simulink model "CM020A_Bmw5441McuCfg"  (R2013b)
settings: Solver=FixedStepDiscrete  SolverMode=SingleTasking  StartTime=0.0  StopTime=1  FixedStep=0.0005  RelTol=1e-3
PreLoadFcn:
  | CM020A_Bmw5441McuCfg_DataDict
values from neighbouring files (symbols this model uses):
  ADC0CFGANDUSE_ADCD0SGVCEP2_CNT_U08 = DataDict.Constant    [CM020A_Bmw5441McuCfg_DataDict.m]
  ADC0CFGANDUSE_ADCD0SGVCEP3_CNT_U08 = DataDict.Constant    [CM020A_Bmw5441McuCfg_DataDict.m]
  ADC0CFGANDUSE_ADCD0SGVCSP2_CNT_U08 = DataDict.Constant    [CM020A_Bmw5441McuCfg_DataDict.m]
  ADC0CFGANDUSE_ADCD0SGVCSP3_CNT_U08 = DataDict.Constant    [CM020A_Bmw5441McuCfg_DataDict.m]
  ADC0CFGANDUSE_ADCD0VCR00_CNT_U32 = DataDict.Constant    [CM020A_Bmw5441McuCfg_DataDict.m]
  ADC0CFGANDUSE_ADCD0VCR01_CNT_U32 = DataDict.Constant    [CM020A_Bmw5441McuCfg_DataDict.m]
  ADC0CFGANDUSE_ADCD0VCR02_CNT_U32 = DataDict.Constant    [CM020A_Bmw5441McuCfg_DataDict.m]
  ADC0CFGANDUSE_ADCD0VCR03_CNT_U32 = DataDict.Constant    [CM020A_Bmw5441McuCfg_DataDict.m]
  ADC0CFGANDUSE_ADCD0VCR04_CNT_U32 = DataDict.Constant    [CM020A_Bmw5441McuCfg_DataDict.m]
  ADC0CFGANDUSE_ADCD0VCR05_CNT_U32 = DataDict.Constant    [CM020A_Bmw5441McuCfg_DataDict.m]
  ADC0CFGANDUSE_ADCD0VCR06_CNT_U32 = DataDict.Constant    [CM020A_Bmw5441McuCfg_DataDict.m]
  ADC0CFGANDUSE_ADCD0VCR07_CNT_U32 = DataDict.Constant    [CM020A_Bmw5441McuCfg_DataDict.m]
  ADC0CFGANDUSE_ADCD0VCR08_CNT_U32 = DataDict.Constant    [CM020A_Bmw5441McuCfg_DataDict.m]
  ADC0CFGANDUSE_ADCD0VCR09_CNT_U32 = DataDict.Constant    [CM020A_Bmw5441McuCfg_DataDict.m]
  ADC0CFGANDUSE_ADCD0VCR10_CNT_U32 = DataDict.Constant    [CM020A_Bmw5441McuCfg_DataDict.m]
  ADC0CFGANDUSE_ADCD0VCR11_CNT_U32 = DataDict.Constant    [CM020A_Bmw5441McuCfg_DataDict.m]
  ADC0CFGANDUSE_ADCD0VCR12_CNT_U32 = DataDict.Constant    [CM020A_Bmw5441McuCfg_DataDict.m]
  ADC0CFGANDUSE_ADCD0VCR13_CNT_U32 = DataDict.Constant    [CM020A_Bmw5441McuCfg_DataDict.m]
  ADC0CFGANDUSE_ADCD0VCR14_CNT_U32 = DataDict.Constant    [CM020A_Bmw5441McuCfg_DataDict.m]
  ADC0CFGANDUSE_ADCD0VCR15_CNT_U32 = DataDict.Constant    [CM020A_Bmw5441McuCfg_DataDict.m]
  ADC0CFGANDUSE_ADCD0VCR16_CNT_U32 = DataDict.Constant    [CM020A_Bmw5441McuCfg_DataDict.m]
  ADC0CFGANDUSE_ADCD0VCR17_CNT_U32 = DataDict.Constant    [CM020A_Bmw5441McuCfg_DataDict.m]
  ADC0CFGANDUSE_ADCD0VCR18_CNT_U32 = DataDict.Constant    [CM020A_Bmw5441McuCfg_DataDict.m]
  ADC0CFGANDUSE_ADCD0VCR19_CNT_U32 = DataDict.Constant    [CM020A_Bmw5441McuCfg_DataDict.m]
  ADC0CFGANDUSE_ADCD0VCR20_CNT_U32 = DataDict.Constant    [CM020A_Bmw5441McuCfg_DataDict.m]
  ADC0CFGANDUSE_ADCSCAGFAC_VOLTPERCNT_F32 = DataDict.Constant    [CM020A_Bmw5441McuCfg_DataDict.m]
  ADC1CFGANDUSE_ADCD1SGVCEP2_CNT_U08 = DataDict.Constant    [CM020A_Bmw5441McuCfg_DataDict.m]
  ADC1CFGANDUSE_ADCD1SGVCEP3_CNT_U08 = DataDict.Constant    [CM020A_Bmw5441McuCfg_DataDict.m]
  ADC1CFGANDUSE_ADCD1SGVCSP2_CNT_U08 = DataDict.Constant    [CM020A_Bmw5441McuCfg_DataDict.m]
  ADC1CFGANDUSE_ADCD1SGVCSP3_CNT_U08 = DataDict.Constant    [CM020A_Bmw5441McuCfg_DataDict.m]
  ADC1CFGANDUSE_ADCD1VCR00_CNT_U32 = DataDict.Constant    [CM020A_Bmw5441McuCfg_DataDict.m]
  ADC1CFGANDUSE_ADCD1VCR01_CNT_U32 = DataDict.Constant    [CM020A_Bmw5441McuCfg_DataDict.m]
  ADC1CFGANDUSE_ADCD1VCR02_CNT_U32 = DataDict.Constant    [CM020A_Bmw5441McuCfg_DataDict.m]
  ADC1CFGANDUSE_ADCD1VCR03_CNT_U32 = DataDict.Constant    [CM020A_Bmw5441McuCfg_DataDict.m]
  ADC1CFGANDUSE_ADCD1VCR04_CNT_U32 = DataDict.Constant    [CM020A_Bmw5441McuCfg_DataDict.m]
  ADC1CFGANDUSE_ADCD1VCR05_CNT_U32 = DataDict.Constant    [CM020A_Bmw5441McuCfg_DataDict.m]
  ADC1CFGANDUSE_ADCD1VCR06_CNT_U32 = DataDict.Constant    [CM020A_Bmw5441McuCfg_DataDict.m]
  ADC1CFGANDUSE_ADCD1VCR07_CNT_U32 = DataDict.Constant    [CM020A_Bmw5441McuCfg_DataDict.m]
  ADC1CFGANDUSE_ADCD1VCR08_CNT_U32 = DataDict.Constant    [CM020A_Bmw5441McuCfg_DataDict.m]
  ADC1CFGANDUSE_ADCD1VCR09_CNT_U32 = DataDict.Constant    [CM020A_Bmw5441McuCfg_DataDict.m]
  ADC1CFGANDUSE_ADCD1VCR10_CNT_U32 = DataDict.Constant    [CM020A_Bmw5441McuCfg_DataDict.m]
  ADC1CFGANDUSE_ADCD1VCR11_CNT_U32 = DataDict.Constant    [CM020A_Bmw5441McuCfg_DataDict.m]
  ADC1CFGANDUSE_ADCD1VCR12_CNT_U32 = DataDict.Constant    [CM020A_Bmw5441McuCfg_DataDict.m]
  ADC1CFGANDUSE_ADCD1VCR13_CNT_U32 = DataDict.Constant    [CM020A_Bmw5441McuCfg_DataDict.m]
  ADC1CFGANDUSE_ADCD1VCR14_CNT_U32 = DataDict.Constant    [CM020A_Bmw5441McuCfg_DataDict.m]
  ADC1CFGANDUSE_ADCD1VCR15_CNT_U32 = DataDict.Constant    [CM020A_Bmw5441McuCfg_DataDict.m]
  ADC1CFGANDUSE_ADCD1VCR16_CNT_U32 = DataDict.Constant    [CM020A_Bmw5441McuCfg_DataDict.m]
  ADC1CFGANDUSE_ADCD1VCR17_CNT_U32 = DataDict.Constant    [CM020A_Bmw5441McuCfg_DataDict.m]
  ADC1CFGANDUSE_ADCD1VCR18_CNT_U32 = DataDict.Constant    [CM020A_Bmw5441McuCfg_DataDict.m]
  ADC1CFGANDUSE_ADCD1VCR19_CNT_U32 = DataDict.Constant    [CM020A_Bmw5441McuCfg_DataDict.m]
  ADC1CFGANDUSE_ADCD1VCR20_CNT_U32 = DataDict.Constant    [CM020A_Bmw5441McuCfg_DataDict.m]
  ADCDIAGC_DYNDIAGFAILSTEP_CNT_U16 = DataDict.Constant    [CM020A_Bmw5441McuCfg_DataDict.m]
  ADCDIAGC_DYNDIAGPASSSTEP_CNT_U16 = DataDict.Constant    [CM020A_Bmw5441McuCfg_DataDict.m]
  BATTRTNCURR_CURRESTIMDIFTHD_AMPR_F32 = DataDict.Constant    [CM020A_Bmw5441McuCfg_DataDict.m]
  BATTRTNCURR_FAILSTEP_CNT_U16 = DataDict.Constant    [CM020A_Bmw5441McuCfg_DataDict.m]
  BATTRTNCURR_FASTLOOPPROC_CNT_LOGL = DataDict.Constant    [CM020A_Bmw5441McuCfg_DataDict.m]
  BATTRTNCURR_FILCUTFREQ_HZ_F32 = DataDict.Constant    [CM020A_Bmw5441McuCfg_DataDict.m]
  BATTRTNCURR_GAIN_AMPRPERVOLT_F32 = DataDict.Constant    [CM020A_Bmw5441McuCfg_DataDict.m]
  BATTRTNCURR_LOWRTHD_AMPR_F32 = DataDict.Constant    [CM020A_Bmw5441McuCfg_DataDict.m]
  BATTRTNCURR_OFFSET_VOLT_F32 = DataDict.Constant    [CM020A_Bmw5441McuCfg_DataDict.m]
  BATTRTNCURR_OUTPMAX_AMPR_F32 = DataDict.Constant    [CM020A_Bmw5441McuCfg_DataDict.m]
  BATTRTNCURR_OUTPMIN_AMPR_F32 = DataDict.Constant    [CM020A_Bmw5441McuCfg_DataDict.m]
  BATTRTNCURR_PASSSTEP_CNT_U16 = DataDict.Constant    [CM020A_Bmw5441McuCfg_DataDict.m]
  BATTRTNCURR_UPPRTHD_AMPR_F32 = DataDict.Constant    [CM020A_Bmw5441McuCfg_DataDict.m]
  BATTVLTGSCAGFAC_ULS_F32 = DataDict.Constant    [CM020A_Bmw5441McuCfg_DataDict.m]
  BATTVLTGSWD1SCAGFAC_ULS_F32 = DataDict.Constant    [CM020A_Bmw5441McuCfg_DataDict.m]
  ECUTMEAS_DFTT_DEGCGRD_F32 = DataDict.Constant    [CM020A_Bmw5441McuCfg_DataDict.m]
  ECUTMEAS_ECUTX_VOLT_U3P13 = DataDict.Constant    [CM020A_Bmw5441McuCfg_DataDict.m]
  ECUTMEAS_ECUTY_DEGCGRD_S8P7 = DataDict.Constant    [CM020A_Bmw5441McuCfg_DataDict.m]
  ECUTMEAS_FILTAU_HZ_F32 = DataDict.Constant    [CM020A_Bmw5441McuCfg_DataDict.m]
  ECUTMEAS_NTC0X045FAILSTEP_CNT_U16 = DataDict.Constant    [CM020A_Bmw5441McuCfg_DataDict.m]
  ECUTMEAS_NTC0X045PASSSTEP_CNT_U16 = DataDict.Constant    [CM020A_Bmw5441McuCfg_DataDict.m]
  ECUTMEAS_RNGDIAGCMAX_DEGCGRD_F32 = DataDict.Constant    [CM020A_Bmw5441McuCfg_DataDict.m]
  ECUTMEAS_RNGDIAGCMIN_DEGCGRD_F32 = DataDict.Constant    [CM020A_Bmw5441McuCfg_DataDict.m]
  ELECGLBPRM_IVTRCNT_CNT_U08 = DataDict.Constant    [CM020A_Bmw5441McuCfg_DataDict.m]
  ELECGLBPRM_PWMFRQMAX_HZ_U32 = DataDict.Constant    [CM020A_Bmw5441McuCfg_DataDict.m]
  ELECGLBPRM_PWMFRQMIN_HZ_U32 = DataDict.Constant    [CM020A_Bmw5441McuCfg_DataDict.m]
  ELECGLBPRM_PWMPERDMAX_NANOSEC_U32 = DataDict.Constant    [CM020A_Bmw5441McuCfg_DataDict.m]
  ELECGLBPRM_PWMPERDMIN_NANOSEC_U32 = DataDict.Constant    [CM020A_Bmw5441McuCfg_DataDict.m]
  ELECGLBPRM_PWMPERDNOM_MICROSEC_U7P9 = DataDict.Constant    [CM020A_Bmw5441McuCfg_DataDict.m]
  ELECGLBPRM_PWMPERDNOMX2_SEC_F32 = DataDict.Constant    [CM020A_Bmw5441McuCfg_DataDict.m]
  FLTINJENA = DataDict.Constant    [CM020A_Bmw5441McuCfg_DataDict.m]
  HWTQ4MEAS_HWTQ4RNGCHKPRTCLNTCNR_CNT_ENUM = DataDict.Constant    [CM020A_Bmw5441McuCfg_DataDict.m]
  HWTQ4MEAS_HWTQ4SCANOTPRFMMFGNTCNR_CNT_ENUM = DataDict.Constant    [CM020A_Bmw5441McuCfg_DataDict.m]
  HWTQ4MEAS_HWTQ4TRIMNOTPRFMMFGNTCNR_CNT_ENUM = DataDict.Constant    [CM020A_Bmw5441McuCfg_DataDict.m]
  HWTQ4MEAS_HWTQBARSTFN_NMPDEG_F32 = DataDict.Constant    [CM020A_Bmw5441McuCfg_DataDict.m]
  HWTQ4MEAS_HWTQOFFS_VOLT_F32 = DataDict.Constant    [CM020A_Bmw5441McuCfg_DataDict.m]
  HWTQ4MEAS_HWTQSNSRSCANOMVAL_VOLTPDEG_F32 = DataDict.Constant    [CM020A_Bmw5441McuCfg_DataDict.m]
  HWTQ5MEAS_HWTQ5RNGCHKPRTCLNTCNR_CNT_ENUM = DataDict.Constant    [CM020A_Bmw5441McuCfg_DataDict.m]
  HWTQ5MEAS_HWTQ5SCANOTPRFMMFGNTCNR_CNT_ENUM = DataDict.Constant    [CM020A_Bmw5441McuCfg_DataDict.m]
  HWTQ5MEAS_HWTQ5TRIMNOTPRFMMFGNTCNR_CNT_ENUM = DataDict.Constant    [CM020A_Bmw5441McuCfg_DataDict.m]
  HWTQ5MEAS_HWTQBARSTFN_NMPDEG_F32 = DataDict.Constant    [CM020A_Bmw5441McuCfg_DataDict.m]
  HWTQ5MEAS_HWTQOFFS_VOLT_F32 = DataDict.Constant    [CM020A_Bmw5441McuCfg_DataDict.m]
  HWTQ5MEAS_HWTQSNSRSCANOMVAL_VOLTPDEG_F32 = DataDict.Constant    [CM020A_Bmw5441McuCfg_DataDict.m]
  MOTAG0MEAS_MOTAG0PRTCLFLTNTCNR_CNT_ENUM = DataDict.Constant    [CM020A_Bmw5441McuCfg_DataDict.m]
  MOTAG1MEAS_MOTAG1PRTCLFLTNTCNR_CNT_ENUM = DataDict.Constant    [CM020A_Bmw5441McuCfg_DataDict.m]
  MOTAG3MEAS_SNSRRLVBITWIDTHEXP_CNT_U08 = DataDict.Constant    [CM020A_Bmw5441McuCfg_DataDict.m]
  MOTAG4MEAS_SNSRRLVBITWIDTHEXP_CNT_U08 = DataDict.Constant    [CM020A_Bmw5441McuCfg_DataDict.m]
  RVSBATTPROTN_FAILSTEP_CNT_U16 = DataDict.Constant    [CM020A_Bmw5441McuCfg_DataDict.m]
  RVSBATTPROTN_GNDMEASDVLTGHILIMN_VOLT_F32 = DataDict.Constant    [CM020A_Bmw5441McuCfg_DataDict.m]
  RVSBATTPROTN_GNDMEASDVLTGLOLIMN_VOLT_F32 = DataDict.Constant    [CM020A_Bmw5441McuCfg_DataDict.m]
  RVSBATTPROTN_PASSSTEP_CNT_U16 = DataDict.Constant    [CM020A_Bmw5441McuCfg_DataDict.m]
  RVSBATTPROTN_RTNMEASDVLTGHILIMN_VOLT_F32 = DataDict.Constant    [CM020A_Bmw5441McuCfg_DataDict.m]
  RVSBATTPROTN_RTNMEASDVLTGLOLIMN_VOLT_F32 = DataDict.Constant    [CM020A_Bmw5441McuCfg_DataDict.m]
  RVSBATTPROTN_RVSFLTTHD_VOLT_F32 = DataDict.Constant    [CM020A_Bmw5441McuCfg_DataDict.m]
  SWPENA = DataDict.Constant    [CM020A_Bmw5441McuCfg_DataDict.m]
  TUNSELNAUTHY_XCPVEHSPDTHD_KPH_F32 = DataDict.Constant    [CM020A_Bmw5441McuCfg_DataDict.m]
libraries: CM020A_Bmw5441McuCfg_ModelLibrary x82, simulink x24
(part 2 of 3)

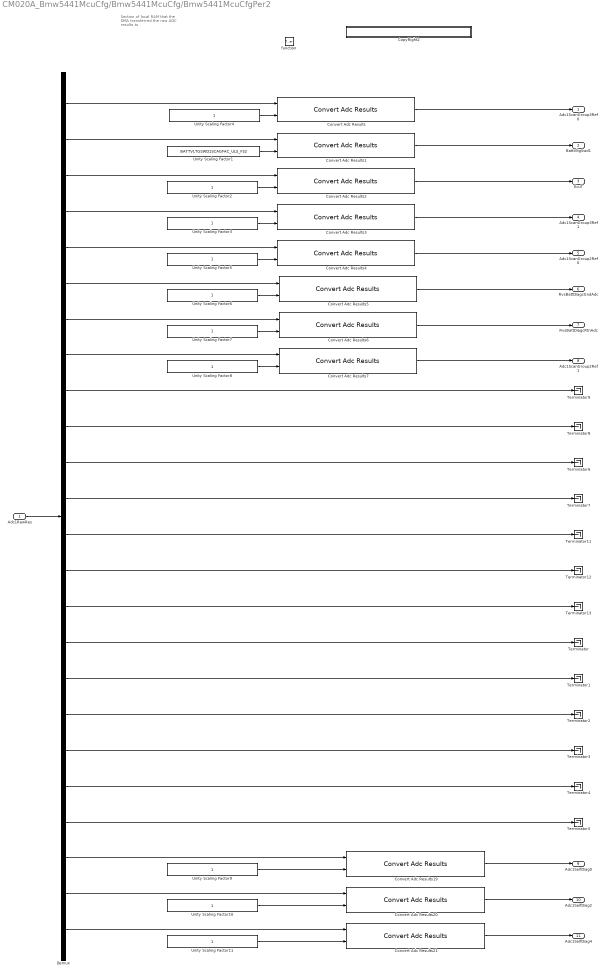
== system CM020A_Bmw5441McuCfg/Bmw5441McuCfg/Bmw5441McuCfgPer2 ==
  note: Section of local RAM that the
      | DMA transferred the raw
      | ADC results to
  Adc1RawRes : Inport
  function : TriggerPort  TriggerType=function-call
  Convert Adc Results{,1..7,19..21} (11 alike) : CM020A_Bmw5441McuCfg_ModelLibrary/Convert Adc Results
  CopyRight2 : Subsystem  Description=|  mask(Copyright Information){none=on}
      | Copyright info block.                                               
      |                                                                     
      | Place copyright information at the top of every subsystem in design.
      mask prompts: none "No parameters"
      mask help: Place copyright information at the top of every subsystem in design.
      mask Display:
      | NxtrConf = 'Nexteer Confidential';
      | 
      | sys = bdroot; %handle for the current model ("system")
      | first = get_param(sys,'Created');
      | first = first(end-3:end);  %year is last four digits
      | 
      | last = get_param(sys,'LastModifiedDate');
      | if isempty(last)
      |     last = datestr(now,'yyyy');
      | else
      |     last = last(end-3:end);
      | end
      | 
      | if strcmp(first,last)
      |     fprintf('%s -- Copyright %s Nexteer',NxtrConf,first)
      | else
      |     fprintf('%s -- %s%s- %s Nexteer',NxtrConf,char(169),first,last)
      | end
  Demux : Demux  Outputs=24
  Terminator{,1..9,11..13} (13 alike) : Terminator
  Unity Scaling Factor1 : Constant  Value=BATTVLTGSWD1SCAGFAC_ULS_F32  OutDataTypeStr=single
  Unity Scaling Factor{2..11} (10 alike) : Constant  OutDataTypeStr=single
  Adc1ScanGroup3Ref0 : Outport
  BattVltgSwd1 : Outport  Port=2
  EcuT : Outport  Port=3
  Adc1ScanGroup3Ref1 : Outport  Port=4
  Adc1ScanGroup2Ref0 : Outport  Port=5
  RvsBattDiagcGndAdc : Outport  Port=6
  RvsBattDiagcRtnAdc : Outport  Port=7
  Adc1ScanGroup2Ref1 : Outport  Port=8
  Adc1SelfDiag0 : Outport  Port=9
  Adc1SelfDiag2 : Outport  Port=10
  Adc1SelfDiag4 : Outport  Port=11
  wires:
  Demux/17 -> Terminator1/1
  Demux/18 -> Terminator2/1
  Demux/19 -> Terminator3/1
  Demux/20 -> Terminator4/1
  Demux/21 -> Terminator5/1
  Demux/16 -> Terminator/1
  Unity Scaling Factor11/1 -> Convert Adc Results21/2
  Demux/24 -> Convert Adc Results21/1
  Unity Scaling Factor10/1 -> Convert Adc Results20/2
  Demux/23 -> Convert Adc Results20/1
  Unity Scaling Factor9/1 -> Convert Adc Results19/2
  Demux/22 -> Convert Adc Results19/1
  Demux/13 -> Terminator11/1
  Demux/14 -> Terminator12/1
  Demux/15 -> Terminator13/1
  Adc1RawRes/1 -> Demux/1
  Demux/5 -> Convert Adc Results4/1
  Unity Scaling Factor3/1 -> Convert Adc Results3/2
  Demux/4 -> Convert Adc Results3/1
  Unity Scaling Factor2/1 -> Convert Adc Results2/2
  Demux/3 -> Convert Adc Results2/1
  Unity Scaling Factor1/1 -> Convert Adc Results1/2
  Demux/2 -> Convert Adc Results1/1
  Demux/1 -> Convert Adc Results/1
  Unity Scaling Factor4/1 -> Convert Adc Results/2
  Demux/10 -> Terminator8/1
  Demux/9 -> Terminator9/1
  Unity Scaling Factor8/1 -> Convert Adc Results7/2
  Demux/8 -> Convert Adc Results7/1
  Unity Scaling Factor7/1 -> Convert Adc Results6/2
  Demux/7 -> Convert Adc Results6/1
  Demux/6 -> Convert Adc Results5/1
  Unity Scaling Factor6/1 -> Convert Adc Results5/2
  Demux/11 -> Terminator6/1
  Demux/12 -> Terminator7/1
  Convert Adc Results/1 -> Adc1ScanGroup3Ref0/1
  Convert Adc Results1/1 -> BattVltgSwd1/1
  Convert Adc Results2/1 -> EcuT/1
  Convert Adc Results3/1 -> Adc1ScanGroup3Ref1/1
  Convert Adc Results4/1 -> Adc1ScanGroup2Ref0/1
  Convert Adc Results5/1 -> RvsBattDiagcGndAdc/1
  Convert Adc Results6/1 -> RvsBattDiagcRtnAdc/1
  Convert Adc Results7/1 -> Adc1ScanGroup2Ref1/1
  Convert Adc Results21/1 -> Adc1SelfDiag4/1
  Convert Adc Results20/1 -> Adc1SelfDiag2/1
  Convert Adc Results19/1 -> Adc1SelfDiag0/1
  Unity Scaling Factor5/1 -> Convert Adc Results4/2

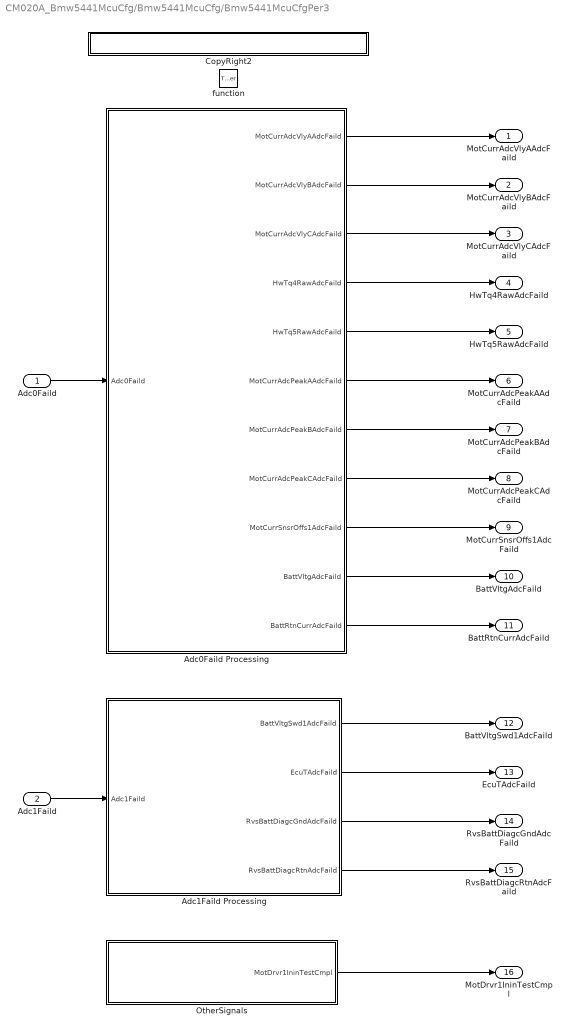
== system CM020A_Bmw5441McuCfg/Bmw5441McuCfg/Bmw5441McuCfgPer3 ==
  Adc0Faild : Inport
  Adc1Faild : Inport  Port=2
  function : TriggerPort  TriggerType=function-call
  Adc0Faild Processing : Subsystem  TreatAsAtomicUnit=on
  Adc1Faild Processing : Subsystem  TreatAsAtomicUnit=on
  CopyRight2 : Subsystem  Description=|  mask(Copyright Information){none=on}
      | Copyright info block.                                               
      |                                                                     
      | Place copyright information at the top of every subsystem in design.
      mask prompts: none "No parameters"
      mask help: Place copyright information at the top of every subsystem in design.
      mask Display:
      | NxtrConf = 'Nexteer Confidential';
      | 
      | sys = bdroot; %handle for the current model ("system")
      | first = get_param(sys,'Created');
      | first = first(end-3:end);  %year is last four digits
      | 
      | last = get_param(sys,'LastModifiedDate');
      | if isempty(last)
      |     last = datestr(now,'yyyy');
      | else
      |     last = last(end-3:end);
      | end
      | 
      | if strcmp(first,last)
      |     fprintf('%s -- Copyright %s Nexteer',NxtrConf,first)
      | else
      |     fprintf('%s -- %s%s- %s Nexteer',NxtrConf,char(169),first,last)
      | end
  OtherSignals : Subsystem  TreatAsAtomicUnit=on
  MotCurrAdcVlyAAdcFaild : Outport
  MotCurrAdcVlyBAdcFaild : Outport  Port=2
  MotCurrAdcVlyCAdcFaild : Outport  Port=3
  HwTq4RawAdcFaild : Outport  Port=4
  HwTq5RawAdcFaild : Outport  Port=5
  MotCurrAdcPeakAAdcFaild : Outport  Port=6
  MotCurrAdcPeakBAdcFaild : Outport  Port=7
  MotCurrAdcPeakCAdcFaild : Outport  Port=8
  MotCurrSnsrOffs1AdcFaild : Outport  Port=9
  BattVltgAdcFaild : Outport  Port=10
  BattRtnCurrAdcFaild : Outport  Port=11
  BattVltgSwd1AdcFaild : Outport  Port=12
  EcuTAdcFaild : Outport  Port=13
  RvsBattDiagcGndAdcFaild : Outport  Port=14
  RvsBattDiagcRtnAdcFaild : Outport  Port=15
  MotDrvr1IninTestCmpl : Outport  Port=16
  wires:
  Adc0Faild/1 -> Adc0Faild Processing/1(Adc0Faild)
  Adc1Faild/1 -> Adc1Faild Processing/1(Adc1Faild)
  Adc1Faild Processing/1(BattVltgSwd1AdcFaild) -> BattVltgSwd1AdcFaild/1
  Adc1Faild Processing/2(EcuTAdcFaild) -> EcuTAdcFaild/1
  Adc0Faild Processing/4(HwTq4RawAdcFaild) -> HwTq4RawAdcFaild/1
  Adc0Faild Processing/5(HwTq5RawAdcFaild) -> HwTq5RawAdcFaild/1
  Adc0Faild Processing/1(MotCurrAdcVlyAAdcFaild) -> MotCurrAdcVlyAAdcFaild/1
  Adc0Faild Processing/2(MotCurrAdcVlyBAdcFaild) -> MotCurrAdcVlyBAdcFaild/1
  Adc0Faild Processing/3(MotCurrAdcVlyCAdcFaild) -> MotCurrAdcVlyCAdcFaild/1
  Adc0Faild Processing/6(MotCurrAdcPeakAAdcFaild) -> MotCurrAdcPeakAAdcFaild/1
  Adc0Faild Processing/7(MotCurrAdcPeakBAdcFaild) -> MotCurrAdcPeakBAdcFaild/1
  Adc0Faild Processing/8(MotCurrAdcPeakCAdcFaild) -> MotCurrAdcPeakCAdcFaild/1
  Adc0Faild Processing/9(MotCurrSnsrOffs1AdcFaild) -> MotCurrSnsrOffs1AdcFaild/1
  Adc0Faild Processing/10(BattVltgAdcFaild) -> BattVltgAdcFaild/1
  Adc0Faild Processing/11(BattRtnCurrAdcFaild) -> BattRtnCurrAdcFaild/1
  Adc1Faild Processing/3(RvsBattDiagcGndAdcFaild) -> RvsBattDiagcGndAdcFaild/1
  Adc1Faild Processing/4(RvsBattDiagcRtnAdcFaild) -> RvsBattDiagcRtnAdcFaild/1
  OtherSignals/1(MotDrvr1IninTestCmpl) -> MotDrvr1IninTestCmpl/1

== system CM020A_Bmw5441McuCfg/Bmw5441McuCfg/CopyRight2 ==

== system CM020A_Bmw5441McuCfg/Bmw5441McuCfg/Bmw5441McuCfgInit1/CopyRight2 ==

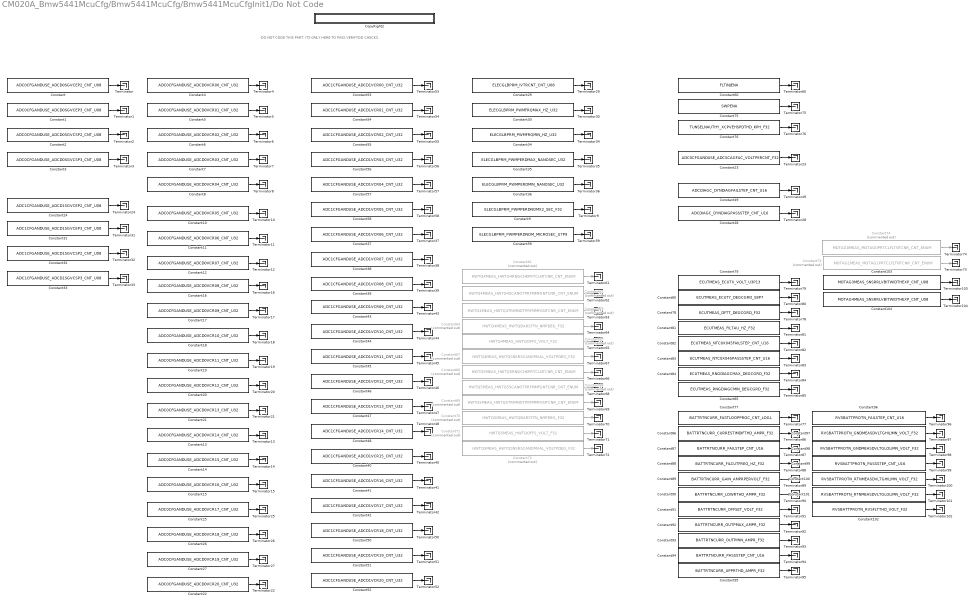
== system CM020A_Bmw5441McuCfg/Bmw5441McuCfg/Bmw5441McuCfgInit1/Do Not Code ==
  note: DO NOT CODE THIS PART.
      | ITS ONLY HERE TO PASS VERIFYDD CHECKS.
  Constant : Constant  Value=ADC0CFGANDUSE_ADCD0SGVCEP2_CNT_U08
  Constant1 : Constant  Value=ADC0CFGANDUSE_ADCD0SGVCEP3_CNT_U08
  Constant10 : Constant  Value=ADC0CFGANDUSE_ADCD0VCR05_CNT_U32
  Constant100 : Constant  Value=RVSBATTPROTN_RTNMEASDVLTGHILIMN_VOLT_F32
  Constant101 : Constant  Value=RVSBATTPROTN_RTNMEASDVLTGLOLIMN_VOLT_F32
  Constant102 : Constant  Value=RVSBATTPROTN_RVSFLTTHD_VOLT_F32
  Constant103 : Constant  Value=MOTAG3MEAS_SNSRRLVBITWIDTHEXP_CNT_U08
  Constant104 : Constant  Value=MOTAG4MEAS_SNSRRLVBITWIDTHEXP_CNT_U08
  Constant11 : Constant  Value=ADC0CFGANDUSE_ADCD0VCR06_CNT_U32
  Constant12 : Constant  Value=ADC0CFGANDUSE_ADCD0VCR07_CNT_U32
  Constant13 : Constant  Value=ADC0CFGANDUSE_ADCD0VCR14_CNT_U32
  Constant14 : Constant  Value=ADC0CFGANDUSE_ADCD0VCR15_CNT_U32
  Constant15 : Constant  Value=ADC0CFGANDUSE_ADCD0VCR16_CNT_U32
  Constant16 : Constant  Value=ADC0CFGANDUSE_ADCD0VCR08_CNT_U32
  Constant17 : Constant  Value=ADC0CFGANDUSE_ADCD0VCR09_CNT_U32
  Constant18 : Constant  Value=ADC0CFGANDUSE_ADCD0VCR10_CNT_U32
  Constant19 : Constant  Value=ADC0CFGANDUSE_ADCD0VCR11_CNT_U32
  Constant2 : Constant  Value=ADC0CFGANDUSE_ADCD0SGVCSP2_CNT_U08
  Constant20 : Constant  Value=ADC0CFGANDUSE_ADCD0VCR12_CNT_U32
  Constant21 : Constant  Value=ADC0CFGANDUSE_ADCD0VCR13_CNT_U32
  Constant22 : Constant  Value=ADC0CFGANDUSE_ADCD0VCR20_CNT_U32
  Constant23 : Constant  Value=ADC0CFGANDUSE_ADCSCAGFAC_VOLTPERCNT_F32
  Constant24 : Constant  Value=ADC1CFGANDUSE_ADCD1SGVCEP2_CNT_U08
  Constant25 : Constant  Value=ADC0CFGANDUSE_ADCD0VCR17_CNT_U32
  Constant26 : Constant  Value=ADC0CFGANDUSE_ADCD0VCR18_CNT_U32
  Constant27 : Constant  Value=ADC0CFGANDUSE_ADCD0VCR19_CNT_U32
  Constant28 : Constant  Value=ADCDIAGC_DYNDIAGPASSSTEP_CNT_U16
  Constant29 : Constant  Value=ELECGLBPRM_IVTRCNT_CNT_U08
  Constant3 : Constant  Value=ADC0CFGANDUSE_ADCD0SGVCSP3_CNT_U08
  Constant30 : Constant  Value=ELECGLBPRM_PWMFRQMAX_HZ_U32
  Constant31 : Constant  Value=ADC1CFGANDUSE_ADCD1SGVCEP3_CNT_U08
  Constant32 : Constant  Value=ADC1CFGANDUSE_ADCD1SGVCSP2_CNT_U08
  Constant33 : Constant  Value=ADC1CFGANDUSE_ADCD1SGVCSP3_CNT_U08
  Constant34 : Constant  Value=ELECGLBPRM_PWMFRQMIN_HZ_U32
  Constant35 : Constant  Value=ELECGLBPRM_PWMPERDMAX_NANOSEC_U32
  Constant36 : Constant  Value=ELECGLBPRM_PWMPERDMIN_NANOSEC_U32
  Constant37 : Constant  Value=ADC1CFGANDUSE_ADCD1VCR06_CNT_U32
  Constant38 : Constant  Value=ADC1CFGANDUSE_ADCD1VCR07_CNT_U32
  Constant39 : Constant  Value=ADC1CFGANDUSE_ADCD1VCR08_CNT_U32
  Constant4 : Constant  Value=ADC0CFGANDUSE_ADCD0VCR00_CNT_U32
  Constant40 : Constant  Value=ADC1CFGANDUSE_ADCD1VCR15_CNT_U32
  Constant41 : Constant  Value=ADC1CFGANDUSE_ADCD1VCR16_CNT_U32
  Constant42 : Constant  Value=ADC1CFGANDUSE_ADCD1VCR17_CNT_U32
  Constant43 : Constant  Value=ADC1CFGANDUSE_ADCD1VCR09_CNT_U32
  Constant44 : Constant  Value=ADC1CFGANDUSE_ADCD1VCR10_CNT_U32
  Constant45 : Constant  Value=ADC1CFGANDUSE_ADCD1VCR11_CNT_U32
  Constant46 : Constant  Value=ADC1CFGANDUSE_ADCD1VCR12_CNT_U32
  Constant47 : Constant  Value=ADC1CFGANDUSE_ADCD1VCR13_CNT_U32
  Constant48 : Constant  Value=ADC1CFGANDUSE_ADCD1VCR14_CNT_U32
  Constant49 : Constant  Value=ADCDIAGC_DYNDIAGFAILSTEP_CNT_U16
  Constant5 : Constant  Value=ADC0CFGANDUSE_ADCD0VCR01_CNT_U32
  Constant50 : Constant  Value=ADC1CFGANDUSE_ADCD1VCR18_CNT_U32
  Constant51 : Constant  Value=ADC1CFGANDUSE_ADCD1VCR19_CNT_U32
  Constant52 : Constant  Value=ADC1CFGANDUSE_ADCD1VCR20_CNT_U32
  Constant53 : Constant  Value=ADC1CFGANDUSE_ADCD1VCR00_CNT_U32
  Constant54 : Constant  Value=ADC1CFGANDUSE_ADCD1VCR01_CNT_U32
  Constant55 : Constant  Value=ADC1CFGANDUSE_ADCD1VCR02_CNT_U32
  Constant56 : Constant  Value=ADC1CFGANDUSE_ADCD1VCR03_CNT_U32
  Constant57 : Constant  Value=ADC1CFGANDUSE_ADCD1VCR04_CNT_U32
  Constant58 : Constant  Value=ADC1CFGANDUSE_ADCD1VCR05_CNT_U32
  Constant59 : Constant  Value=ELECGLBPRM_PWMPERDNOM_MICROSEC_U7P9
  Constant6 : Constant  Value=ADC0CFGANDUSE_ADCD0VCR02_CNT_U32
  Constant60 : Constant  Value=FLTINJENA
  Constant61 : Constant  Commented=on  Value=HWTQ4MEAS_HWTQ4RNGCHKPRTCLNTCNR_CNT_ENUM
  Constant62 : Constant  Commented=on  Value=HWTQ4MEAS_HWTQ4SCANOTPRFMMFGNTCNR_CNT_ENUM
  Constant63 : Constant  Commented=on  Value=HWTQ4MEAS_HWTQ4TRIMNOTPRFMMFGNTCNR_CNT_ENUM
  Constant64 : Constant  Commented=on  Value=HWTQ4MEAS_HWTQBARSTFN_NMPDEG_F32
  Constant65 : Constant  Commented=on  Value=HWTQ4MEAS_HWTQOFFS_VOLT_F32
  Constant66 : Constant  Commented=on  Value=HWTQ5MEAS_HWTQ5RNGCHKPRTCLNTCNR_CNT_ENUM
  Constant67 : Constant  Commented=on  Value=HWTQ4MEAS_HWTQSNSRSCANOMVAL_VOLTPDEG_F32
  Constant68 : Constant  Commented=on  Value=HWTQ5MEAS_HWTQ5SCANOTPRFMMFGNTCNR_CNT_ENUM
  Constant69 : Constant  Commented=on  Value=HWTQ5MEAS_HWTQ5TRIMNOTPRFMMFGNTCNR_CNT_ENUM
  Constant7 : Constant  Value=ADC0CFGANDUSE_ADCD0VCR03_CNT_U32
  Constant70 : Constant  Commented=on  Value=HWTQ5MEAS_HWTQBARSTFN_NMPDEG_F32
  Constant71 : Constant  Commented=on  Value=HWTQ5MEAS_HWTQOFFS_VOLT_F32
  Constant72 : Constant  Commented=on  Value=HWTQ5MEAS_HWTQSNSRSCANOMVAL_VOLTPDEG_F32
  Constant73 : Constant  Commented=on  Value=MOTAG1MEAS_MOTAG1PRTCLFLTNTCNR_CNT_ENUM
  Constant74 : Constant  Commented=on  Value=MOTAG0MEAS_MOTAG0PRTCLFLTNTCNR_CNT_ENUM
  Constant75 : Constant  Value=SWPENA
  Constant76 : Constant  Value=TUNSELNAUTHY_XCPVEHSPDTHD_KPH_F32
  Constant77 : Constant  Value=BATTRTNCURR_FASTLOOPPROC_CNT_LOGL
  Constant78 : Constant  Value=ECUTMEAS_DFTT_DEGCGRD_F32
  Constant79 : Constant  Value=ECUTMEAS_ECUTX_VOLT_U3P13
  Constant8 : Constant  Value=ADC0CFGANDUSE_ADCD0VCR04_CNT_U32
  Constant80 : Constant  Value=ECUTMEAS_ECUTY_DEGCGRD_S8P7
  Constant81 : Constant  Value=ECUTMEAS_FILTAU_HZ_F32
  Constant82 : Constant  Value=ECUTMEAS_NTC0X045FAILSTEP_CNT_U16
  Constant83 : Constant  Value=ECUTMEAS_NTC0X045PASSSTEP_CNT_U16
  Constant84 : Constant  Value=ECUTMEAS_RNGDIAGCMAX_DEGCGRD_F32
  Constant85 : Constant  Value=ECUTMEAS_RNGDIAGCMIN_DEGCGRD_F32
  Constant86 : Constant  Value=BATTRTNCURR_CURRESTIMDIFTHD_AMPR_F32
  Constant87 : Constant  Value=BATTRTNCURR_FAILSTEP_CNT_U16
  Constant88 : Constant  Value=BATTRTNCURR_FILCUTFREQ_HZ_F32
  Constant89 : Constant  Value=BATTRTNCURR_GAIN_AMPRPERVOLT_F32
  Constant9 : Constant  Value=ELECGLBPRM_PWMPERDNOMX2_SEC_F32
  Constant90 : Constant  Value=BATTRTNCURR_LOWRTHD_AMPR_F32
  Constant91 : Constant  Value=BATTRTNCURR_OFFSET_VOLT_F32
  Constant92 : Constant  Value=BATTRTNCURR_OUTPMAX_AMPR_F32
  Constant93 : Constant  Value=BATTRTNCURR_OUTPMIN_AMPR_F32
  Constant94 : Constant  Value=BATTRTNCURR_PASSSTEP_CNT_U16
  Constant95 : Constant  Value=BATTRTNCURR_UPPRTHD_AMPR_F32
  Constant96 : Constant  Value=RVSBATTPROTN_FAILSTEP_CNT_U16
  Constant97 : Constant  Value=RVSBATTPROTN_GNDMEASDVLTGHILIMN_VOLT_F32
  Constant98 : Constant  Value=RVSBATTPROTN_GNDMEASDVLTGLOLIMN_VOLT_F32
  Constant99 : Constant  Value=RVSBATTPROTN_PASSSTEP_CNT_U16
  CopyRight2 : Subsystem  Description=|  mask(Copyright Information){none=on}
      | Copyright info block.                                               
      |                                                                     
      | Place copyright information at the top of every subsystem in design.
      mask prompts: none "No parameters"
      mask help: Place copyright information at the top of every subsystem in design.
      mask Display:
      | NxtrConf = 'Nexteer Confidential';
      | 
      | sys = bdroot; %handle for the current model ("system")
      | first = get_param(sys,'Created');
      | first = first(end-3:end);  %year is last four digits
      | 
      | last = get_param(sys,'LastModifiedDate');
      | if isempty(last)
      |     last = datestr(now,'yyyy');
      | else
      |     last = last(end-3:end);
      | end
      | 
      | if strcmp(first,last)
      |     fprintf('%s -- Copyright %s Nexteer',NxtrConf,first)
      | else
      |     fprintf('%s -- %s%s- %s Nexteer',NxtrConf,char(169),first,last)
      | end
  Terminator{,1..104} (105 alike) : Terminator
  wires:
  Constant/1 -> Terminator/1
  Constant1/1 -> Terminator1/1
  Constant2/1 -> Terminator2/1
  Constant3/1 -> Terminator3/1
  Constant4/1 -> Terminator4/1
  Constant5/1 -> Terminator5/1
  Constant6/1 -> Terminator6/1
  Constant7/1 -> Terminator7/1
  Constant8/1 -> Terminator8/1
  Constant10/1 -> Terminator10/1
  Constant11/1 -> Terminator11/1
  Constant12/1 -> Terminator12/1
  Constant16/1 -> Terminator16/1
  Constant17/1 -> Terminator17/1
  Constant18/1 -> Terminator18/1
  Constant19/1 -> Terminator19/1
  Constant20/1 -> Terminator20/1
  Constant21/1 -> Terminator21/1
  Constant13/1 -> Terminator13/1
  Constant14/1 -> Terminator14/1
  Constant15/1 -> Terminator15/1
  Constant25/1 -> Terminator25/1
  Constant26/1 -> Terminator26/1
  Constant27/1 -> Terminator27/1
  Constant22/1 -> Terminator22/1
  Constant23/1 -> Terminator23/1
  Constant24/1 -> Terminator24/1
  Constant31/1 -> Terminator31/1
  Constant32/1 -> Terminator32/1
  Constant33/1 -> Terminator33/1
  Constant28/1 -> Terminator28/1
  Constant29/1 -> Terminator29/1
  Constant30/1 -> Terminator30/1
  Constant34/1 -> Terminator34/1
  Constant35/1 -> Terminator35/1
  Constant36/1 -> Terminator36/1
  Constant53/1 -> Terminator53/1
  Constant54/1 -> Terminator54/1
  Constant55/1 -> Terminator55/1
  Constant56/1 -> Terminator56/1
  Constant57/1 -> Terminator57/1
  Constant58/1 -> Terminator58/1
  Constant37/1 -> Terminator37/1
  Constant38/1 -> Terminator38/1
  Constant39/1 -> Terminator39/1
  Constant43/1 -> Terminator43/1
  Constant44/1 -> Terminator44/1
  Constant45/1 -> Terminator45/1
  Constant46/1 -> Terminator46/1
  Constant47/1 -> Terminator47/1
  Constant48/1 -> Terminator48/1
  Constant40/1 -> Terminator40/1
  Constant41/1 -> Terminator41/1
  Constant42/1 -> Terminator42/1
  Constant50/1 -> Terminator50/1
  Constant51/1 -> Terminator51/1
  Constant52/1 -> Terminator52/1
  Constant49/1 -> Terminator49/1
  Constant9/1 -> Terminator9/1
  Constant59/1 -> Terminator59/1
  Constant60/1 -> Terminator60/1
  Constant61/1 -> Terminator61/1
  Constant62/1 -> Terminator62/1
  Constant63/1 -> Terminator63/1
  Constant64/1 -> Terminator64/1
  Constant65/1 -> Terminator65/1
  Constant67/1 -> Terminator67/1
  Constant66/1 -> Terminator66/1
  Constant68/1 -> Terminator68/1
  Constant69/1 -> Terminator69/1
  Constant70/1 -> Terminator70/1
  Constant71/1 -> Terminator71/1
  Constant72/1 -> Terminator72/1
  Constant74/1 -> Terminator74/1
  Constant73/1 -> Terminator73/1
  Constant75/1 -> Terminator75/1
  Constant76/1 -> Terminator76/1
  Constant77/1 -> Terminator77/1
  Constant78/1 -> Terminator78/1
  Constant79/1 -> Terminator79/1
  Constant80/1 -> Terminator80/1
  Constant81/1 -> Terminator81/1
  Constant82/1 -> Terminator82/1
  Constant83/1 -> Terminator83/1
  Constant84/1 -> Terminator84/1
  Constant85/1 -> Terminator85/1
  Constant86/1 -> Terminator86/1
  Constant87/1 -> Terminator87/1
  Constant88/1 -> Terminator88/1
  Constant89/1 -> Terminator89/1
  Constant90/1 -> Terminator90/1
  Constant91/1 -> Terminator91/1
  Constant92/1 -> Terminator92/1
  Constant93/1 -> Terminator93/1
  Constant94/1 -> Terminator94/1
  Constant95/1 -> Terminator95/1
  Constant96/1 -> Terminator96/1
  Constant97/1 -> Terminator97/1
  Constant98/1 -> Terminator98/1
  Constant99/1 -> Terminator99/1
  Constant100/1 -> Terminator100/1
  Constant101/1 -> Terminator101/1
  Constant102/1 -> Terminator102/1
  Constant103/1 -> Terminator103/1
  Constant104/1 -> Terminator104/1

== system CM020A_Bmw5441McuCfg/Bmw5441McuCfg/Bmw5441McuCfgInit1/Register Initialization ==
  note: Bmw5441McuCfg Configuration
      |
      |     Order by row
      |
      | 1. Initialize Digital Noise Filter Registers According to DigitalNoiseFilterConfig.xlsx. Please note delays after Enabling DNF (see Rational below).
      | 2. Initialize PortConfig According to CM020A_Bmw5441McuCfg_PortConfig.xlsm.
      | 3. Initialize the PIC2B registers from the following sources in the order listed:
      | 	1. Run Adc0CfgAndUseInit1 - this means to run the AdcCfgInit function first before this init function, there is no client or server call
      | 		IMPORTANT - update ADCD1VCR00 - ADCD1VCR23 and Virtual Channel configuration according to CM020A_Bmw5441McuCfg_AdcConfig.xlsm
      | 	2  Run Adc1CfgAndUseInit1 - this means to run the AdcCfgInit function first before this init function, there is no client or server call
      | 		IMPORTANT - update ADCD0VCR00 - ADCD0VCR23 and Virtual Channel configuration according to CM020A_Bmw5441McuCfg_AdcConfig.xlsm
      | 	3. CM020A_Bmw5441McuCfg_RegisterConfiguration.xlsm
  note: Rational for 12 cycles Delay in DigitalNoiseFilterConfig.xlsx:
      |
      | According to datasheet "Notes for Digital Noise Filter":
      | When digital filter output signal is input for alternative function, enable the digital filter and switch the port pin to
      | alternative function after a lapse of the following time:
      |
      | Time = s × 1/fs + 2 × 1/DNFATCKI
      | Where s = DNFAnNFSTS[1:0] + 2.
      |
      | Configuration:
      | DNFAnFSTS is configured for 2 samples.
      | DNFATCKI is CLK_HSB (80MHz)
      | DNFAnPRS is configured for sampling frequency (DNFATCKI / 1), therfore fs = DNFATCKI/1 = CLK_HSB.
      |
      | Time = 4/CLK_HSB + 2/CLK_HSB = 6/CLK_HSB.
      |
      | CLK_HSB is 80MHz, where CPU clock (CLK_CPU) is 160MHz, therefore we need 12 cycles.
  CopyRight2 : Subsystem  Description=|  mask(Copyright Information){none=on}
      | Copyright info block.                                               
      |                                                                     
      | Place copyright information at the top of every subsystem in design.
      mask prompts: none "No parameters"
      mask help: Place copyright information at the top of every subsystem in design.
      mask Display:
      | NxtrConf = 'Nexteer Confidential';
      | 
      | sys = bdroot; %handle for the current model ("system")
      | first = get_param(sys,'Created');
      | first = first(end-3:end);  %year is last four digits
      | 
      | last = get_param(sys,'LastModifiedDate');
      | if isempty(last)
      |     last = datestr(now,'yyyy');
      | else
      |     last = last(end-3:end);
      | end
      | 
      | if strcmp(first,last)
      |     fprintf('%s -- Copyright %s Nexteer',NxtrConf,first)
      | else
      |     fprintf('%s -- %s%s- %s Nexteer',NxtrConf,char(169),first,last)
      | end

== system CM020A_Bmw5441McuCfg/Bmw5441McuCfg/Bmw5441McuCfgInit2/CopyRight2 ==

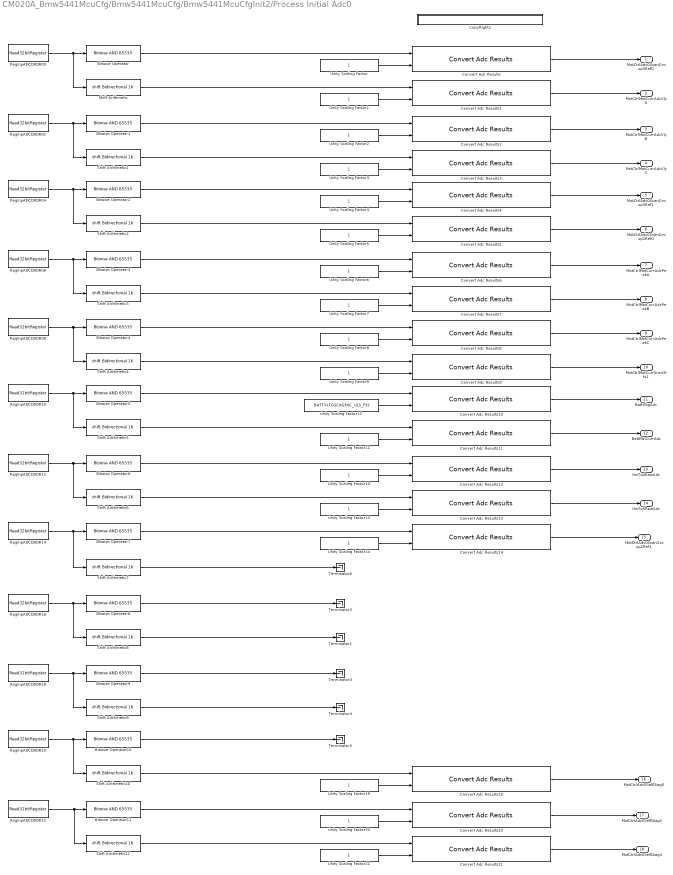
== system CM020A_Bmw5441McuCfg/Bmw5441McuCfg/Bmw5441McuCfgInit2/Process Initial Adc0 ==
  Bitwise Operator{,1..11} (12 alike) : simulink/Logic and Bit Operations/Bitwise Operator  logicop=AND  UseBitMask=on  BitMask=65535  BitMaskRealWorld=Stored Integer
  Convert Adc Results{,1..14,19..21} (18 alike) : CM020A_Bmw5441McuCfg_ModelLibrary/Convert Adc Results
  CopyRight2 : Subsystem  Description=|  mask(Copyright Information){none=on}
      | Copyright info block.                                               
      |                                                                     
      | Place copyright information at the top of every subsystem in design.
      mask prompts: none "No parameters"
      mask help: Place copyright information at the top of every subsystem in design.
      mask Display:
      | NxtrConf = 'Nexteer Confidential';
      | 
      | sys = bdroot; %handle for the current model ("system")
      | first = get_param(sys,'Created');
      | first = first(end-3:end);  %year is last four digits
      | 
      | last = get_param(sys,'LastModifiedDate');
      | if isempty(last)
      |     last = datestr(now,'yyyy');
      | else
      |     last = last(end-3:end);
      | end
      | 
      | if strcmp(first,last)
      |     fprintf('%s -- Copyright %s Nexteer',NxtrConf,first)
      | else
      |     fprintf('%s -- %s%s- %s Nexteer',NxtrConf,char(169),first,last)
      | end
  RegInpADCD0DR00 : CM020A_Bmw5441McuCfg_ModelLibrary/Read32bitRegister
  RegInpADCD0DR02 : CM020A_Bmw5441McuCfg_ModelLibrary/Read32bitRegister
  RegInpADCD0DR04 : CM020A_Bmw5441McuCfg_ModelLibrary/Read32bitRegister
  RegInpADCD0DR06 : CM020A_Bmw5441McuCfg_ModelLibrary/Read32bitRegister
  RegInpADCD0DR08 : CM020A_Bmw5441McuCfg_ModelLibrary/Read32bitRegister
  RegInpADCD0DR{10,12,14,16,18,20,22} (7 alike) : CM020A_Bmw5441McuCfg_ModelLibrary/Read32bitRegister
  Shift Arithmetic{,1..11} (12 alike) : ArithShift  BitShiftNumber=16
  Terminator{1..6} (6 alike) : Terminator
  Unity Scaling Factor{,1..11,13..14,19..21} (17 alike) : Constant  OutDataTypeStr=single
  Unity Scaling Factor12 : Constant  Value=BATTVLTGSCAGFAC_ULS_F32  OutDataTypeStr=single
  MotCtrlAdc0ScanGroup3Ref0 : Outport
  MotCtrlMotCurrAdcVlyA : Outport  Port=2
  MotCtrlMotCurrAdcVlyB : Outport  Port=3
  MotCtrlMotCurrAdcVlyC : Outport  Port=4
  MotCtrlAdc0ScanGroup3Ref1 : Outport  Port=5
  MotCtrlAdc0ScanGroup2Ref0 : Outport  Port=6
  MotCtrlMotCurrAdcPeakA : Outport  Port=7
  MotCtrlMotCurrAdcPeakB : Outport  Port=8
  MotCtrlMotCurrAdcPeakC : Outport  Port=9
  MotCtrlMotCurrSnsrOffs1 : Outport  Port=10
  BattVltgAdc : Outport  Port=11
  BattRtnCurrAdc : Outport  Port=12
  HwTq4RawAdc : Outport  Port=13
  HwTq5RawAdc : Outport  Port=14
  MotCtrlAdc0ScanGroup2Ref1 : Outport  Port=15
  MotCtrlAdc0SelfDiag0 : Outport  Port=16
  MotCtrlAdc0SelfDiag2 : Outport  Port=17
  MotCtrlAdc0SelfDiag4 : Outport  Port=18
  wires:
  Bitwise Operator/1 -> Convert Adc Results/1
  Unity Scaling Factor/1 -> Convert Adc Results/2
  Shift Arithmetic/1 -> Convert Adc Results1/1
  Unity Scaling Factor1/1 -> Convert Adc Results1/2
  Unity Scaling Factor2/1 -> Convert Adc Results2/2
  Unity Scaling Factor3/1 -> Convert Adc Results3/2
  Unity Scaling Factor4/1 -> Convert Adc Results4/2
  Unity Scaling Factor5/1 -> Convert Adc Results5/2
  Unity Scaling Factor6/1 -> Convert Adc Results6/2
  Unity Scaling Factor7/1 -> Convert Adc Results7/2
  Unity Scaling Factor8/1 -> Convert Adc Results8/2
  Unity Scaling Factor19/1 -> Convert Adc Results19/2
  Convert Adc Results/1 -> MotCtrlAdc0ScanGroup3Ref0/1
  Convert Adc Results1/1 -> MotCtrlMotCurrAdcVlyA/1
  Convert Adc Results2/1 -> MotCtrlMotCurrAdcVlyB/1
  Convert Adc Results19/1 -> MotCtrlAdc0SelfDiag0/1
  RegInpADCD0DR00/1 -> Bitwise Operator/1, Shift Arithmetic/1
  RegInpADCD0DR02/1 -> Bitwise Operator1/1, Shift Arithmetic1/1
  Bitwise Operator1/1 -> Convert Adc Results2/1
  Shift Arithmetic1/1 -> Convert Adc Results3/1
  RegInpADCD0DR04/1 -> Bitwise Operator2/1, Shift Arithmetic2/1
  RegInpADCD0DR06/1 -> Bitwise Operator3/1, Shift Arithmetic3/1
  RegInpADCD0DR08/1 -> Bitwise Operator4/1, Shift Arithmetic4/1
  RegInpADCD0DR10/1 -> Bitwise Operator5/1, Shift Arithmetic5/1
  RegInpADCD0DR12/1 -> Bitwise Operator6/1, Shift Arithmetic6/1
  RegInpADCD0DR14/1 -> Bitwise Operator7/1, Shift Arithmetic7/1
  RegInpADCD0DR16/1 -> Bitwise Operator8/1, Shift Arithmetic8/1
  RegInpADCD0DR18/1 -> Bitwise Operator9/1, Shift Arithmetic9/1
  Shift Arithmetic10/1 -> Convert Adc Results19/1
  Bitwise Operator10/1 -> Terminator5/1
  Bitwise Operator9/1 -> Terminator3/1
  Shift Arithmetic9/1 -> Terminator4/1
  Bitwise Operator4/1 -> Convert Adc Results8/1
  Bitwise Operator3/1 -> Convert Adc Results6/1
  Shift Arithmetic3/1 -> Convert Adc Results7/1
  Bitwise Operator2/1 -> Convert Adc Results4/1
  Shift Arithmetic2/1 -> Convert Adc Results5/1
  Convert Adc Results3/1 -> MotCtrlMotCurrAdcVlyC/1
  Unity Scaling Factor9/1 -> Convert Adc Results9/2
  Unity Scaling Factor11/1 -> Convert Adc Results11/2
  Unity Scaling Factor13/1 -> Convert Adc Results13/2
  Shift Arithmetic4/1 -> Convert Adc Results9/1
  Bitwise Operator7/1 -> Convert Adc Results14/1
  Bitwise Operator6/1 -> Convert Adc Results12/1
  Shift Arithmetic6/1 -> Convert Adc Results13/1
  Bitwise Operator5/1 -> Convert Adc Results10/1
  Shift Arithmetic5/1 -> Convert Adc Results11/1
  Shift Arithmetic8/1 -> Terminator1/1
  Shift Arithmetic7/1 -> Terminator6/1
  Bitwise Operator8/1 -> Terminator2/1
  Unity Scaling Factor14/1 -> Convert Adc Results14/2
  Unity Scaling Factor20/1 -> Convert Adc Results20/2
  Unity Scaling Factor21/1 -> Convert Adc Results21/2
  Convert Adc Results20/1 -> MotCtrlAdc0SelfDiag2/1
  Convert Adc Results21/1 -> MotCtrlAdc0SelfDiag4/1
  Shift Arithmetic11/1 -> Convert Adc Results21/1
  Bitwise Operator11/1 -> Convert Adc Results20/1
  RegInpADCD0DR20/1 -> Bitwise Operator10/1, Shift Arithmetic10/1
  Convert Adc Results12/1 -> HwTq4RawAdc/1
  Convert Adc Results13/1 -> HwTq5RawAdc/1
  Convert Adc Results14/1 -> MotCtrlAdc0ScanGroup2Ref1/1
  Convert Adc Results11/1 -> BattRtnCurrAdc/1
  Convert Adc Results10/1 -> BattVltgAdc/1
  Convert Adc Results9/1 -> MotCtrlMotCurrSnsrOffs1/1
  Convert Adc Results8/1 -> MotCtrlMotCurrAdcPeakC/1
  Convert Adc Results7/1 -> MotCtrlMotCurrAdcPeakB/1
  Convert Adc Results6/1 -> MotCtrlMotCurrAdcPeakA/1
  Convert Adc Results5/1 -> MotCtrlAdc0ScanGroup2Ref0/1
  Convert Adc Results4/1 -> MotCtrlAdc0ScanGroup3Ref1/1
  Unity Scaling Factor12/1 -> Convert Adc Results10/2
  Unity Scaling Factor10/1 -> Convert Adc Results12/2
  RegInpADCD0DR22/1 -> Shift Arithmetic11/1, Bitwise Operator11/1

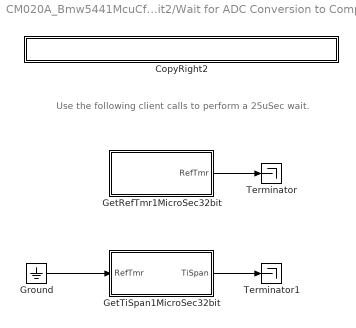
== system CM020A_Bmw5441McuCfg/Bmw5441McuCfg/Bmw5441McuCfgInit2/Wait for ADC Conversion to Complete ==
  note: Use the following client calls to perform a 25uSec wait.
  CopyRight2 : Subsystem  Description=|  mask(Copyright Information){none=on}
      | Copyright info block.                                               
      |                                                                     
      | Place copyright information at the top of every subsystem in design.
      mask prompts: none "No parameters"
      mask help: Place copyright information at the top of every subsystem in design.
      mask Display:
      | NxtrConf = 'Nexteer Confidential';
      | 
      | sys = bdroot; %handle for the current model ("system")
      | first = get_param(sys,'Created');
      | first = first(end-3:end);  %year is last four digits
      | 
      | last = get_param(sys,'LastModifiedDate');
      | if isempty(last)
      |     last = datestr(now,'yyyy');
      | else
      |     last = last(end-3:end);
      | end
      | 
      | if strcmp(first,last)
      |     fprintf('%s -- Copyright %s Nexteer',NxtrConf,first)
      | else
      |     fprintf('%s -- %s%s- %s Nexteer',NxtrConf,char(169),first,last)
      | end
  GetRefTmr1MicroSec32bit : Subsystem  TreatAsAtomicUnit=on
  GetTiSpan1MicroSec32bit : Subsystem  TreatAsAtomicUnit=on
  Ground : Ground
  Terminator : Terminator
  Terminator1 : Terminator
  wires:
  GetRefTmr1MicroSec32bit/1(RefTmr) -> Terminator/1
  GetTiSpan1MicroSec32bit/1(TiSpan) -> Terminator1/1
  Ground/1 -> GetTiSpan1MicroSec32bit/1(RefTmr)

== system CM020A_Bmw5441McuCfg/Bmw5441McuCfg/Bmw5441McuCfgInit3/CopyRight2 ==

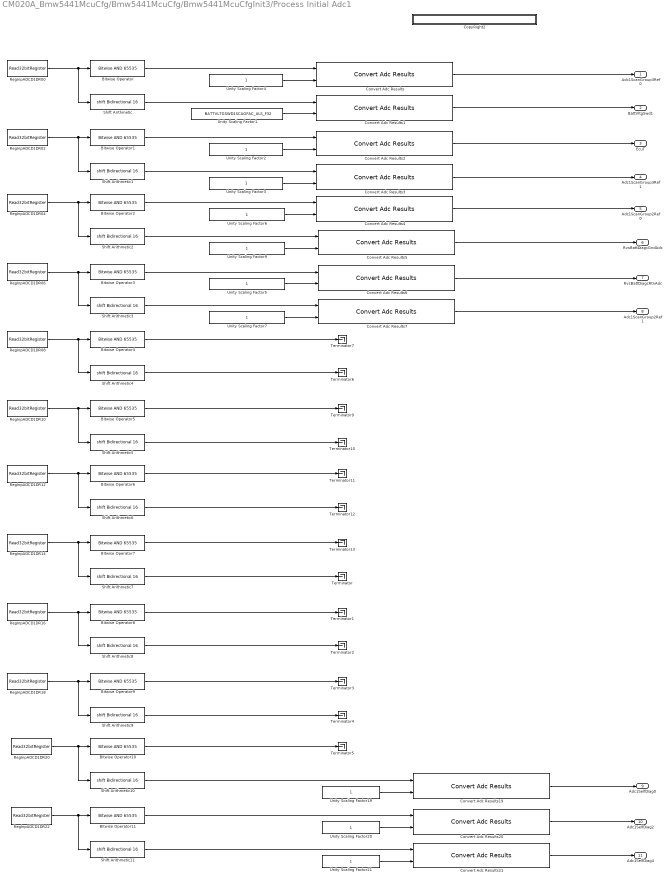
== system CM020A_Bmw5441McuCfg/Bmw5441McuCfg/Bmw5441McuCfgInit3/Process Initial Adc1 ==
  Bitwise Operator{,1..11} (12 alike) : simulink/Logic and Bit Operations/Bitwise Operator  logicop=AND  UseBitMask=on  BitMask=65535  BitMaskRealWorld=Stored Integer
  Convert Adc Results{,1..7,19..21} (11 alike) : CM020A_Bmw5441McuCfg_ModelLibrary/Convert Adc Results
  CopyRight2 : Subsystem  Description=|  mask(Copyright Information){none=on}
      | Copyright info block.                                               
      |                                                                     
      | Place copyright information at the top of every subsystem in design.
      mask prompts: none "No parameters"
      mask help: Place copyright information at the top of every subsystem in design.
      mask Display:
      | NxtrConf = 'Nexteer Confidential';
      | 
      | sys = bdroot; %handle for the current model ("system")
      | first = get_param(sys,'Created');
      | first = first(end-3:end);  %year is last four digits
      | 
      | last = get_param(sys,'LastModifiedDate');
      | if isempty(last)
      |     last = datestr(now,'yyyy');
      | else
      |     last = last(end-3:end);
      | end
      | 
      | if strcmp(first,last)
      |     fprintf('%s -- Copyright %s Nexteer',NxtrConf,first)
      | else
      |     fprintf('%s -- %s%s- %s Nexteer',NxtrConf,char(169),first,last)
      | end
  RegInpADCD1DR00 : CM020A_Bmw5441McuCfg_ModelLibrary/Read32bitRegister
  RegInpADCD1DR02 : CM020A_Bmw5441McuCfg_ModelLibrary/Read32bitRegister
  RegInpADCD1DR04 : CM020A_Bmw5441McuCfg_ModelLibrary/Read32bitRegister
  RegInpADCD1DR06 : CM020A_Bmw5441McuCfg_ModelLibrary/Read32bitRegister
  RegInpADCD1DR08 : CM020A_Bmw5441McuCfg_ModelLibrary/Read32bitRegister
  RegInpADCD1DR{10,12,14,16,18,20,22} (7 alike) : CM020A_Bmw5441McuCfg_ModelLibrary/Read32bitRegister
  Shift Arithmetic{,1..11} (12 alike) : ArithShift  BitShiftNumber=16
  Terminator{,1..7,9..13} (13 alike) : Terminator
  Unity Scaling Factor1 : Constant  Value=BATTVLTGSWD1SCAGFAC_ULS_F32  OutDataTypeStr=single
  Unity Scaling Factor{2..7,9,19..21} (10 alike) : Constant  OutDataTypeStr=single
  Adc1ScanGroup3Ref0 : Outport
  BattVltgSwd1 : Outport  Port=2
  EcuT : Outport  Port=3
  Adc1ScanGroup3Ref1 : Outport  Port=4
  Adc1ScanGroup2Ref0 : Outport  Port=5
  RvsBattDiagcGndAdc : Outport  Port=6
  RvsBattDiagcRtnAdc : Outport  Port=7
  Adc1ScanGroup2Ref1 : Outport  Port=8
  Adc1SelfDiag0 : Outport  Port=9
  Adc1SelfDiag2 : Outport  Port=10
  Adc1SelfDiag4 : Outport  Port=11
  wires:
  Convert Adc Results21/1 -> Adc1SelfDiag4/1
  Convert Adc Results20/1 -> Adc1SelfDiag2/1
  Convert Adc Results19/1 -> Adc1SelfDiag0/1
  Unity Scaling Factor21/1 -> Convert Adc Results21/2
  Unity Scaling Factor20/1 -> Convert Adc Results20/2
  Unity Scaling Factor19/1 -> Convert Adc Results19/2
  RegInpADCD1DR00/1 -> Bitwise Operator/1, Shift Arithmetic/1
  RegInpADCD1DR02/1 -> Bitwise Operator1/1, Shift Arithmetic1/1
  RegInpADCD1DR04/1 -> Bitwise Operator2/1, Shift Arithmetic2/1
  RegInpADCD1DR06/1 -> Bitwise Operator3/1, Shift Arithmetic3/1
  RegInpADCD1DR08/1 -> Bitwise Operator4/1, Shift Arithmetic4/1
  RegInpADCD1DR10/1 -> Bitwise Operator5/1, Shift Arithmetic5/1
  RegInpADCD1DR12/1 -> Bitwise Operator6/1, Shift Arithmetic6/1
  RegInpADCD1DR14/1 -> Bitwise Operator7/1, Shift Arithmetic7/1
  RegInpADCD1DR16/1 -> Bitwise Operator8/1, Shift Arithmetic8/1
  RegInpADCD1DR18/1 -> Bitwise Operator9/1, Shift Arithmetic9/1
  RegInpADCD1DR20/1 -> Shift Arithmetic10/1, Bitwise Operator10/1
  RegInpADCD1DR22/1 -> Shift Arithmetic11/1, Bitwise Operator11/1
  Shift Arithmetic11/1 -> Convert Adc Results21/1
  Bitwise Operator11/1 -> Convert Adc Results20/1
  Shift Arithmetic10/1 -> Convert Adc Results19/1
  Bitwise Operator10/1 -> Terminator5/1
  Bitwise Operator9/1 -> Terminator3/1
  Shift Arithmetic9/1 -> Terminator4/1
  Bitwise Operator8/1 -> Terminator1/1
  Shift Arithmetic8/1 -> Terminator2/1
  Shift Arithmetic7/1 -> Terminator/1
  Bitwise Operator5/1 -> Terminator9/1
  Shift Arithmetic5/1 -> Terminator10/1
  Bitwise Operator6/1 -> Terminator11/1
  Shift Arithmetic6/1 -> Terminator12/1
  Bitwise Operator7/1 -> Terminator13/1
  Bitwise Operator2/1 -> Convert Adc Results4/1
  Unity Scaling Factor3/1 -> Convert Adc Results3/2
  Shift Arithmetic1/1 -> Convert Adc Results3/1
  Unity Scaling Factor2/1 -> Convert Adc Results2/2
  Bitwise Operator1/1 -> Convert Adc Results2/1
  Unity Scaling Factor1/1 -> Convert Adc Results1/2
  Shift Arithmetic/1 -> Convert Adc Results1/1
  Bitwise Operator/1 -> Convert Adc Results/1
  Convert Adc Results/1 -> Adc1ScanGroup3Ref0/1
  Unity Scaling Factor4/1 -> Convert Adc Results/2
  Convert Adc Results1/1 -> BattVltgSwd1/1
  Convert Adc Results2/1 -> EcuT/1
  Convert Adc Results3/1 -> Adc1ScanGroup3Ref1/1
  Unity Scaling Factor6/1 -> Convert Adc Results4/2
  Convert Adc Results4/1 -> Adc1ScanGroup2Ref0/1
  Shift Arithmetic4/1 -> Terminator6/1
  Bitwise Operator4/1 -> Terminator7/1
  Unity Scaling Factor7/1 -> Convert Adc Results7/2
  Shift Arithmetic3/1 -> Convert Adc Results7/1
  Unity Scaling Factor5/1 -> Convert Adc Results6/2
  Bitwise Operator3/1 -> Convert Adc Results6/1
  Shift Arithmetic2/1 -> Convert Adc Results5/1
  Convert Adc Results5/1 -> RvsBattDiagcGndAdc/1
  Unity Scaling Factor9/1 -> Convert Adc Results5/2
  Convert Adc Results6/1 -> RvsBattDiagcRtnAdc/1
  Convert Adc Results7/1 -> Adc1ScanGroup2Ref1/1

== system CM020A_Bmw5441McuCfg/Bmw5441McuCfg/Bmw5441McuCfgPer1/CopyRight2 ==

== system CM020A_Bmw5441McuCfg/Bmw5441McuCfg/Bmw5441McuCfgPer2/CopyRight2 ==

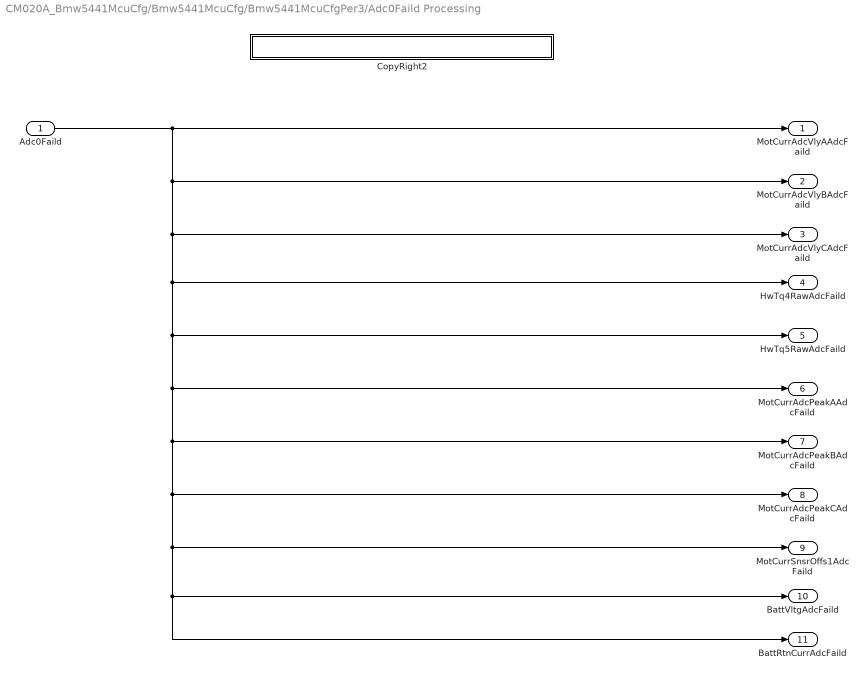
== system CM020A_Bmw5441McuCfg/Bmw5441McuCfg/Bmw5441McuCfgPer3/Adc0Faild Processing ==
  Adc0Faild : Inport
  CopyRight2 : Subsystem  Description=|  mask(Copyright Information){none=on}
      | Copyright info block.                                               
      |                                                                     
      | Place copyright information at the top of every subsystem in design.
      mask prompts: none "No parameters"
      mask help: Place copyright information at the top of every subsystem in design.
      mask Display:
      | NxtrConf = 'Nexteer Confidential';
      | 
      | sys = bdroot; %handle for the current model ("system")
      | first = get_param(sys,'Created');
      | first = first(end-3:end);  %year is last four digits
      | 
      | last = get_param(sys,'LastModifiedDate');
      | if isempty(last)
      |     last = datestr(now,'yyyy');
      | else
      |     last = last(end-3:end);
      | end
      | 
      | if strcmp(first,last)
      |     fprintf('%s -- Copyright %s Nexteer',NxtrConf,first)
      | else
      |     fprintf('%s -- %s%s- %s Nexteer',NxtrConf,char(169),first,last)
      | end
  MotCurrAdcVlyAAdcFaild : Outport
  MotCurrAdcVlyBAdcFaild : Outport  Port=2
  MotCurrAdcVlyCAdcFaild : Outport  Port=3
  HwTq4RawAdcFaild : Outport  Port=4
  HwTq5RawAdcFaild : Outport  Port=5
  MotCurrAdcPeakAAdcFaild : Outport  Port=6
  MotCurrAdcPeakBAdcFaild : Outport  Port=7
  MotCurrAdcPeakCAdcFaild : Outport  Port=8
  MotCurrSnsrOffs1AdcFaild : Outport  Port=9
  BattVltgAdcFaild : Outport  Port=10
  BattRtnCurrAdcFaild : Outport  Port=11
  wires:
  Adc0Faild/1 -> MotCurrAdcVlyAAdcFaild/1, MotCurrAdcVlyBAdcFaild/1, MotCurrAdcVlyCAdcFaild/1, BattRtnCurrAdcFaild/1, BattVltgAdcFaild/1, MotCurrSnsrOffs1AdcFaild/1, MotCurrAdcPeakCAdcFaild/1, MotCurrAdcPeakBAdcFaild/1, MotCurrAdcPeakAAdcFaild/1, HwTq5RawAdcFaild/1, HwTq4RawAdcFaild/1

== system CM020A_Bmw5441McuCfg/Bmw5441McuCfg/Bmw5441McuCfgPer3/Adc1Faild Processing ==
  Adc1Faild : Inport
  CopyRight2 : Subsystem  Description=|  mask(Copyright Information){none=on}
      | Copyright info block.                                               
      |                                                                     
      | Place copyright information at the top of every subsystem in design.
      mask prompts: none "No parameters"
      mask help: Place copyright information at the top of every subsystem in design.
      mask Display:
      | NxtrConf = 'Nexteer Confidential';
      | 
      | sys = bdroot; %handle for the current model ("system")
      | first = get_param(sys,'Created');
      | first = first(end-3:end);  %year is last four digits
      | 
      | last = get_param(sys,'LastModifiedDate');
      | if isempty(last)
      |     last = datestr(now,'yyyy');
      | else
      |     last = last(end-3:end);
      | end
      | 
      | if strcmp(first,last)
      |     fprintf('%s -- Copyright %s Nexteer',NxtrConf,first)
      | else
      |     fprintf('%s -- %s%s- %s Nexteer',NxtrConf,char(169),first,last)
      | end
  BattVltgSwd1AdcFaild : Outport
  EcuTAdcFaild : Outport  Port=2
  RvsBattDiagcGndAdcFaild : Outport  Port=3
  RvsBattDiagcRtnAdcFaild : Outport  Port=4
  wires:
  Adc1Faild/1 -> RvsBattDiagcRtnAdcFaild/1, RvsBattDiagcGndAdcFaild/1, EcuTAdcFaild/1, BattVltgSwd1AdcFaild/1

== system CM020A_Bmw5441McuCfg/Bmw5441McuCfg/Bmw5441McuCfgPer3/CopyRight2 ==
